simulink model "Simulacao"  (Simulink 8.2)
settings: Solver=ode4  SolverMode=SingleTasking  StartTime=0.0  StopTime=20  FixedStep=0.01  RelTol=1e-3
InitFcn:
  | PreLoad;
undefined symbols (not defined in the file or in its folder): A1, B1, C, D, T, xk0
undefined symbols (not defined in the file): A, B, R, S, Umax
settings Model: Creator=Kawakami  LastModifiedBy=Eduardo
settings DataIOCC: LimitDataPoints=off  SaveOutput=off  SaveTime=off  TimeSaveName=t  SignalLoggingName=sigsOut
settings OptimizationCC: BooleanDataType=off
settings DebuggingCC: SaveWithParameterizedLinksMsg=none  SignalResolutionControl=TryResolveAllWithWarning  SolverPrmCheckMsg=none  MultiTaskDSMMsg=warning  MultiTaskCondExecSysMsg=none
settings HardwareCC: TargetUnknown=on
settings RTWCC: IncludeERTFirstTime=on

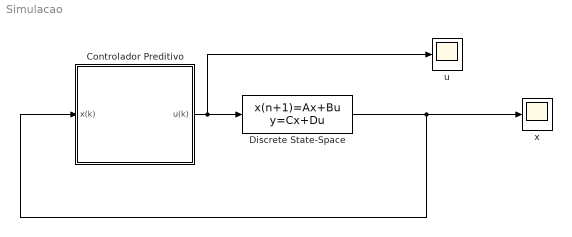
== system Simulacao ==
  "Controlador Preditivo  " : Subsystem  mask{A=A, B=B, S=S, R=R, Umax=Umax, T=T}
      mask prompts: A "Matriz Agregada A"; B "Matriz Agregada B"; S "S (custo quadrático)"; R "R (custo quadrático)"; Umax "Input Max"; T "T (passo da simulação)"
  Discrete State-Space : DiscreteStateSpace  A=A1  B=B1  C=C  D=D  X0=xk0
  u : Scope
      settings: TimeRange=10  YMin=-2  YMax=0.5
  x : Scope
      settings: YMin=-1.25  YMax=2.25
  wires:
  "Controlador Preditivo  "/1(u(k)) -> Discrete State-Space/1, u/1
  Discrete State-Space/1 -> "Controlador Preditivo  "/1(x(k)), x/1

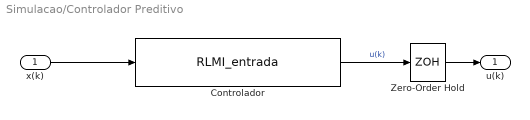
== system Simulacao/Controlador Preditivo   ==
  x(k) : Inport
  Controlador : S-Function  FunctionName=RLMI_entrada  Parameters=S, R, A, B, Umax, T  EnableBusSupport=off
  Zero-Order Hold : ZeroOrderHold  SampleTime=T
  u(k) : Outport
  wires:
  Zero-Order Hold/1 -> u(k)/1
  Controlador/1 -> Zero-Order Hold/1  "u(k)"
  x(k)/1 -> Controlador/1
